simulink model "DOF4_model"  (R2024b)
settings: Solver=FixedStepAuto  StartTime=0.0  StopTime=100  FixedStep=0.005  RelTol=1e-3
values from neighbouring files (symbols this model uses):
  a = 1.8    [DOF4_model_parameters.m]
  b = L-a    (= 1.7)    [DOF4_model_parameters.m]
  cfdamper = 2870    [DOF4_model_parameters.m]
  crdamper = 2540    [DOF4_model_parameters.m]
  F0f = 3740    [DOF4_model_parameters.m]
  F0r = 3960    [DOF4_model_parameters.m]
  g = 9.81    [DOF4_model_parameters.m]
  I = 1350    [DOF4_model_parameters.m]
  kfspring = 135000    [DOF4_model_parameters.m]
  krspring = 100000    [DOF4_model_parameters.m]
  ktyre = 400000    [DOF4_model_parameters.m]
  ms = 785    [DOF4_model_parameters.m]
  musf = 30    [DOF4_model_parameters.m]
  musr = 35    [DOF4_model_parameters.m]
  z0ftyre = (ms*b/L+musf)*g/ktyre    (= 0.0100867821429)    [DOF4_model_parameters.m]
  z0rtyre = (ms*a/L+musr)*g/ktyre    (= 0.0107594678571)    [DOF4_model_parameters.m]
libraries: simulink x1
settings Model: Creator=jayku  LastModifiedBy=jayku

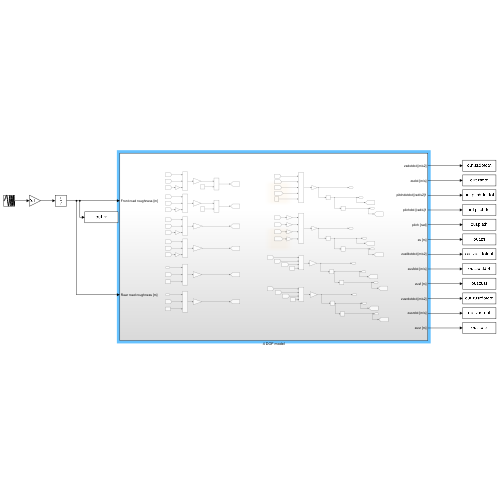
[thumbnail: Simulink's stored preview of the top-level diagram]
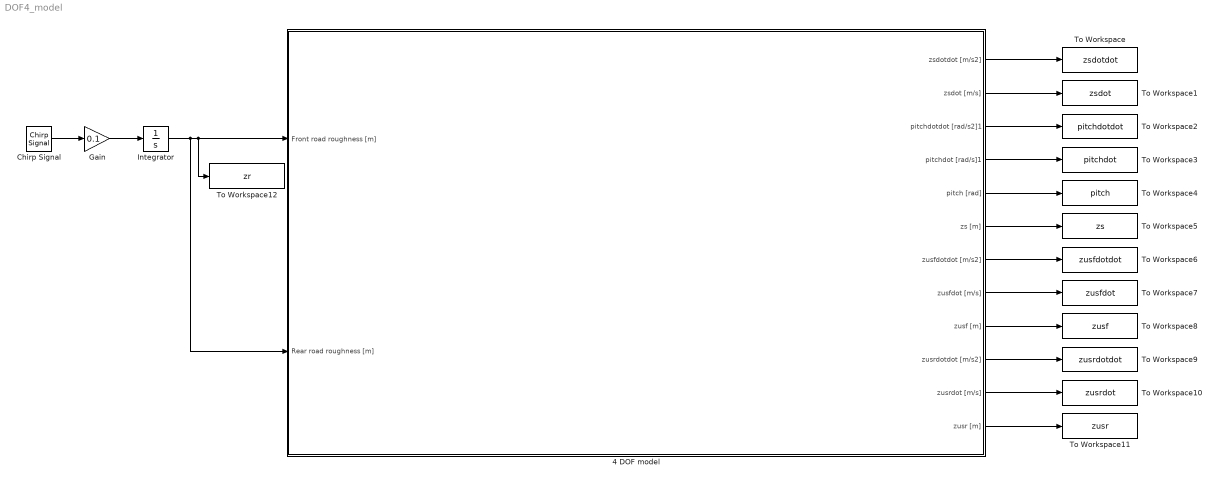
== system DOF4_model ==
  4 DOF model : Subsystem
  Chirp Signal : simulink/Sources/Chirp Signal  f1=0.1  T=100  f2=50
  Gain : Gain  Gain=0.1
  Integrator : Integrator
  To Workspace : ToWorkspace  VariableName=zsdotdot  SaveFormat=Timeseries  SampleTime=-1
  To Workspace1 : ToWorkspace  VariableName=zsdot  SaveFormat=Timeseries  SampleTime=-1
  To Workspace10 : ToWorkspace  VariableName=zusrdot  SaveFormat=Timeseries  SampleTime=-1
  To Workspace11 : ToWorkspace  VariableName=zusr  SaveFormat=Timeseries  SampleTime=-1
  To Workspace12 : ToWorkspace  VariableName=zr  SaveFormat=Timeseries  SampleTime=-1
  To Workspace2 : ToWorkspace  VariableName=pitchdotdot  SaveFormat=Timeseries  SampleTime=-1
  To Workspace3 : ToWorkspace  VariableName=pitchdot  SaveFormat=Timeseries  SampleTime=-1
  To Workspace4 : ToWorkspace  VariableName=pitch  SaveFormat=Timeseries  SampleTime=-1
  To Workspace5 : ToWorkspace  VariableName=zs  SaveFormat=Timeseries  SampleTime=-1
  To Workspace6 : ToWorkspace  VariableName=zusfdotdot  SaveFormat=Timeseries  SampleTime=-1
  To Workspace7 : ToWorkspace  VariableName=zusfdot  SaveFormat=Timeseries  SampleTime=-1
  To Workspace8 : ToWorkspace  VariableName=zusf  SaveFormat=Timeseries  SampleTime=-1
  To Workspace9 : ToWorkspace  VariableName=zusrdotdot  SaveFormat=Timeseries  SampleTime=-1
  wires:
  4 DOF model/1(zsdotdot [m/s2]) -> To Workspace/1
  4 DOF model/2(zsdot [m/s]) -> To Workspace1/1
  4 DOF model/3(pitchdotdot [rad/s2]1) -> To Workspace2/1
  4 DOF model/4(pitchdot [rad/s]1) -> To Workspace3/1
  4 DOF model/5(pitch [rad]) -> To Workspace4/1
  4 DOF model/6(zs [m]) -> To Workspace5/1
  4 DOF model/7(zusfdotdot [m/s2]) -> To Workspace6/1
  4 DOF model/8(zusfdot [m/s]) -> To Workspace7/1
  4 DOF model/9(zusf [m]) -> To Workspace8/1
  4 DOF model/10(zusrdotdot [m/s2]) -> To Workspace9/1
  4 DOF model/11(zusrdot [m/s]) -> To Workspace10/1
  4 DOF model/12(zusr [m]) -> To Workspace11/1
  Chirp Signal/1 -> Gain/1
  Gain/1 -> Integrator/1
  Integrator/1 -> 4 DOF model/2(Rear road roughness [m]), 4 DOF model/1(Front road roughness [m]), To Workspace12/1

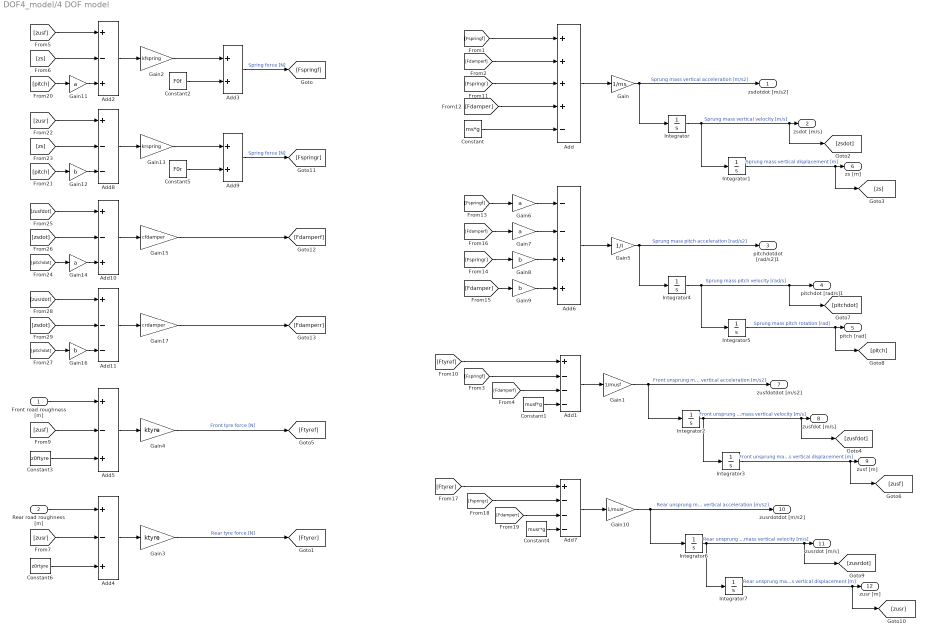
== system DOF4_model/4 DOF model ==
  Front road roughness [m] : Inport
  Rear road roughness [m] : Inport  Port=2
  Add : Sum  Inputs=++++-
  Add1 : Sum  Inputs=+---
  Add{2,4..5,10} (4 alike) : Sum  Inputs=+-+
  Add11 : Sum  Inputs=+--
  Add3 : Sum
  Add6 : Sum  Inputs=--++
  Add7 : Sum  Inputs=+---
  Add8 : Sum  Inputs=+--
  Add9 : Sum
  Constant : Constant  Value=ms*g
  Constant1 : Constant  Value=musf*g
  Constant2 : Constant  Value=F0f
  Constant3 : Constant  Value=z0ftyre
  Constant4 : Constant  Value=musr*g
  Constant5 : Constant  Value=F0r
  Constant6 : Constant  Value=z0rtyre
  Gain : Gain  Gain=1/ms
  Gain1 : Gain  Gain=1/musf
  Gain10 : Gain  Gain=1/musr
  Gain{6..7,11,14} (4 alike) : Gain  Gain=a
  Gain{8..9,12,16} (4 alike) : Gain  Gain=b
  Gain13 : Gain  Gain=krspring
  Gain15 : Gain  Gain=cfdamper
  Gain17 : Gain  Gain=crdamper
  Gain2 : Gain  Gain=kfspring
  Gain3 : Gain  Gain=ktyre
  Gain4 : Gain  Gain=ktyre
  Gain5 : Gain  Gain=1/I
  Integrator{,1..7} (8 alike) : Integrator
  zsdotdot [m/s2] : Outport
  zsdot [m/s] : Outport  Port=2
  pitchdotdot [rad/s2]1 : Outport  Port=3
  pitchdot [rad/s]1 : Outport  Port=4
  pitch [rad] : Outport  Port=5
  zs [m] : Outport  Port=6
  zusfdotdot [m/s2] : Outport  Port=7
  zusfdot [m/s] : Outport  Port=8
  zusf [m] : Outport  Port=9
  zusrdotdot [m/s2] : Outport  Port=10
  zusrdot [m/s] : Outport  Port=11
  zusr [m] : Outport  Port=12
  wires:
  Add1/1 -> Gain1/1
  [Ftyref] -> Add1/1
  Constant3/1 -> Add5/3
  [Fspringf] -> Add1/2
  [Fdamperf] -> Add/2
  Gain2/1 -> Add3/1
  Gain1/1 -> zusfdotdot [m/s2]/1, Integrator2/1  "Front unsprung mass vertical acceleration [m/s2]"
  [Fdamperf] -> Add1/3
  [Fspringf] -> Add/1
  [zusf] -> Add5/2
  Add/1 -> Gain/1
  Integrator3/1 -> [zusf], zusf [m]/1  "Front unsprung mass vertical displacement [m]"
  Integrator2/1 -> [zusfdot], zusfdot [m/s]/1, Integrator3/1  "Front unsprung mass vertical velocity [m/s]"
  Front road roughness [m]/1 -> Add5/1
  Add5/1 -> Gain4/1
  Constant1/1 -> Add1/4
  [zusf] -> Add2/1
  Integrator/1 -> [zsdot], zsdot [m/s]/1, Integrator1/1  "Sprung mass vertical velocity [m/s]"
  Constant/1 -> Add/5
  Gain4/1 -> [Ftyref]  "Front tyre force [N]"
  Gain/1 -> zsdotdot [m/s2]/1, Integrator/1  "Sprung mass vertical acceleration [m/s2]"
  Integrator1/1 -> [zs], zs [m]/1  "Sprung mass vertical displacement [m]"
  Add3/1 -> [Fspringf]  "Spring force [N]"
  [zs] -> Add2/2
  Constant2/1 -> Add3/2
  Add2/1 -> Gain2/1
  [Fspringr] -> Add/3
  [Fdamper] -> Add/4
  [Fdamper] -> Gain9/1
  [Fspringr] -> Gain8/1
  Integrator5/1 -> [pitch], pitch [rad]/1  "Sprung mass pitch rotation [rad]"
  Integrator4/1 -> [pitchdot], pitchdot [rad/s]1/1, Integrator5/1  "Sprung mass pitch velocity [rad/s]"
  [Fdamperf] -> Gain7/1
  [Fspringf] -> Gain6/1
  Gain5/1 -> Integrator4/1, pitchdotdot [rad/s2]1/1  "Sprung mass pitch acceleration [rad/s2]"
  Add6/1 -> Gain5/1
  Gain6/1 -> Add6/1
  Gain7/1 -> Add6/2
  Gain8/1 -> Add6/3
  Gain9/1 -> Add6/4
  Constant4/1 -> Add7/4
  Integrator6/1 -> Integrator7/1, zusrdot [m/s]/1, [zusrdot]  "Rear unsprung mass vertical velocity [m/s]"
  Integrator7/1 -> zusr [m]/1, [zusr]  "Rear unsprung mass vertical displacement [m]"
  [Fdamperr] -> Add7/3
  Gain10/1 -> Integrator6/1, zusrdotdot [m/s2]/1  "Rear unsprung mass vertical acceleration [m/s2]"
  [Fspringr] -> Add7/2
  [Ftyrer] -> Add7/1
  Add7/1 -> Gain10/1
  [pitch] -> Gain11/1
  Gain11/1 -> Add2/3
  Gain12/1 -> Add8/3
  [pitch] -> Gain12/1
  Add8/1 -> Gain13/1
  Constant5/1 -> Add9/2
  [zs] -> Add8/2
  Add9/1 -> [Fspringr]  "Spring force [N]"
  [zusr] -> Add8/1
  Gain13/1 -> Add9/1
  Gain14/1 -> Add10/3
  [pitchdot] -> Gain14/1
  Add10/1 -> Gain15/1
  [zsdot] -> Add10/2
  [zusfdot] -> Add10/1
  Gain15/1 -> [Fdamperf]
  Gain17/1 -> [Fdamperr]
  [zusrdot] -> Add11/1
  [zsdot] -> Add11/2
  Add11/1 -> Gain17/1
  [pitchdot] -> Gain16/1
  Gain16/1 -> Add11/3
  Gain3/1 -> [Ftyrer]  "Rear tyre force [N]"
  Add4/1 -> Gain3/1
  Rear road roughness [m]/1 -> Add4/1
  [zusr] -> Add4/2
  Constant6/1 -> Add4/3
